simulink model "HW4ThrusterModel"  (R2022b)
settings: Solver=VariableStepAuto  StartTime=0.0  StopTime=20.0  RelTol=1e-3
undefined symbols (not defined in the file or in its folder): sat, trigger, trigger2
settings Model: Creator=gagandeepthapar  LastModifiedBy=gagandeepthapar

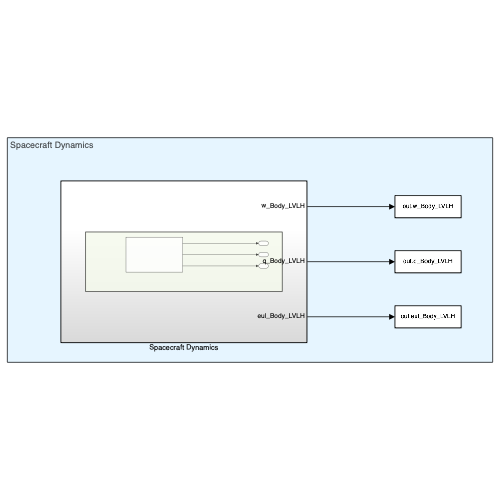
[thumbnail: Simulink's stored preview of the top-level diagram]
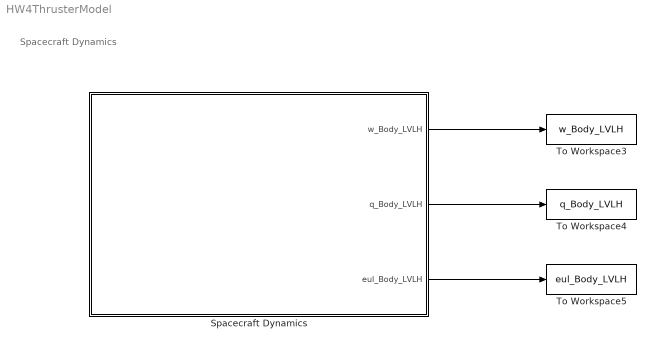
== system HW4ThrusterModel ==
  note: Spacecraft Dynamics
  Spacecraft Dynamics : Subsystem
  To Workspace3 : ToWorkspace  VariableName=w_Body_LVLH  SampleTime=-1
      settings: Save2DSignal=2-D array (concatenate along first dimension)
  To Workspace4 : ToWorkspace  VariableName=q_Body_LVLH  SampleTime=-1
      settings: Save2DSignal=2-D array (concatenate along first dimension)
  To Workspace5 : ToWorkspace  VariableName=eul_Body_LVLH  SampleTime=-1
      settings: Save2DSignal=2-D array (concatenate along first dimension)
  wires:
  Spacecraft Dynamics/1(w_Body_LVLH) -> To Workspace3/1
  Spacecraft Dynamics/2(q_Body_LVLH) -> To Workspace4/1
  Spacecraft Dynamics/3(eul_Body_LVLH) -> To Workspace5/1

== system HW4ThrusterModel/Spacecraft Dynamics ==
  note: Body_LVLH
  Body_LVLH : Subsystem
  w_Body_LVLH : Outport
  q_Body_LVLH : Outport  Port=2
  eul_Body_LVLH : Outport  Port=3
  wires:
  Body_LVLH/1(w_Body_LVLH) -> w_Body_LVLH/1
  Body_LVLH/2(q_Body_LVLH) -> q_Body_LVLH/1
  Body_LVLH/3(eul_Body_LVLH) -> eul_Body_LVLH/1

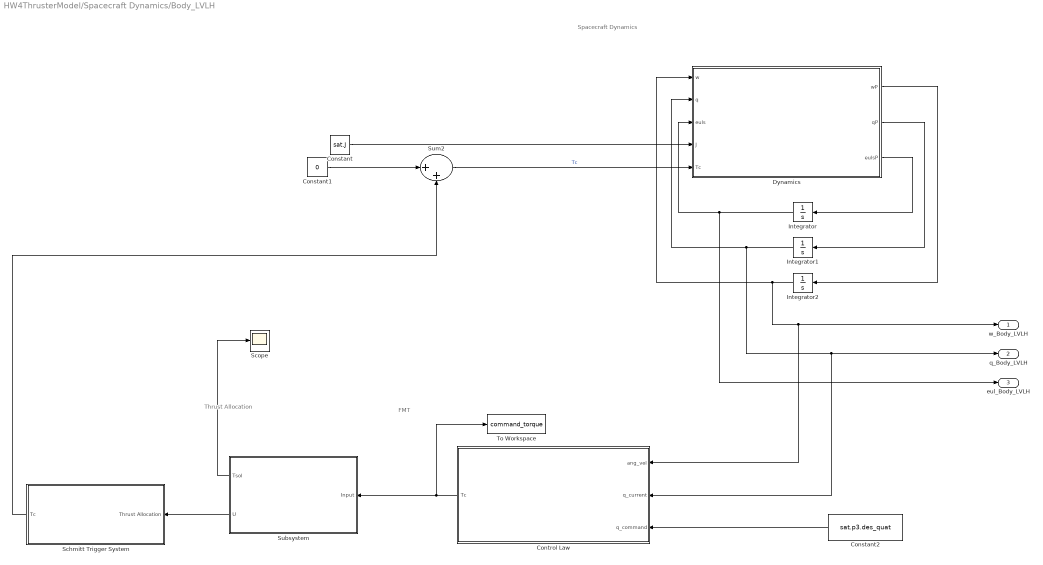
== system HW4ThrusterModel/Spacecraft Dynamics/Body_LVLH ==
  note: Thrust Allocation
  note: Spacecraft Dynamics
  note: FMT
  Constant : Constant  Value=sat.J
  Constant1 : Constant  Value=0
  Constant2 : Constant  Value=sat.p3.des_quat
  Control Law : Subsystem
  Dynamics : MATLAB Function  TreatAsAtomicUnit=on
  Integrator : Integrator  InitialCondition=sat.p3.euls0_lvlh
  Integrator1 : Integrator  InitialCondition=sat.p3.quat0
  Integrator2 : Integrator  InitialCondition=sat.p3.w0_lvlh
  Schmitt Trigger System : Subsystem
  Scope : Scope
  Subsystem : Subsystem
  Sum2 : Sum  Inputs=|++
  To Workspace : ToWorkspace  VariableName=command_torque  SampleTime=-1
      settings: Save2DSignal=2-D array (concatenate along first dimension)
  w_Body_LVLH : Outport
  q_Body_LVLH : Outport  Port=2
  eul_Body_LVLH : Outport  Port=3
  wires:
  Dynamics/3(eulsP) -> Integrator/1
  Dynamics/2(qP) -> Integrator1/1
  Dynamics/1(wP) -> Integrator2/1
  Integrator/1 -> eul_Body_LVLH/1, Dynamics/3(euls)
  Integrator1/1 -> q_Body_LVLH/1, Control Law/2(q_current), Dynamics/2(q)
  Constant/1 -> Dynamics/4(J)
  Constant1/1 -> Sum2/1
  Integrator2/1 -> w_Body_LVLH/1, Control Law/1(ang_vel), Dynamics/1(w)
  Sum2/1 -> Dynamics/5(Tc)  "Tc"
  Control Law/1(Tc) -> To Workspace/1, Subsystem/1(Input)
  Constant2/1 -> Control Law/3(q_command)
  Subsystem/2(U) -> Schmitt Trigger System/1(Thrust Allocation)
  Subsystem/1(Tsol) -> Scope/1
  Schmitt Trigger System/1(Tc) -> Sum2/2

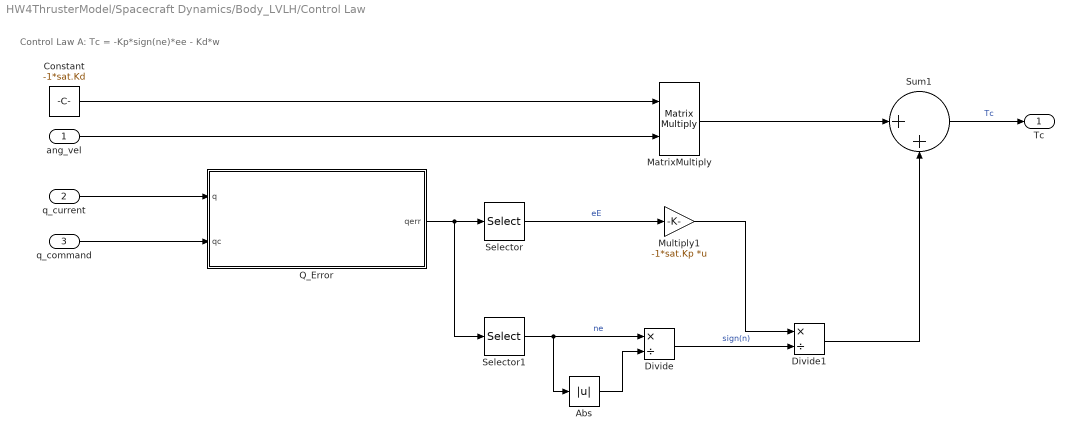
== system HW4ThrusterModel/Spacecraft Dynamics/Body_LVLH/Control Law ==
  note: Control Law A: Tc = -Kp*sign(ne)*ee - Kd*w
  ang_vel : Inport
  q_current : Inport  Port=2
  q_command : Inport  Port=3
  Abs : Abs  SaturateOnIntegerOverflow=off
  Constant : Constant  Value=-1*sat.Kd
  Divide : Product  Inputs=*/
  Divide1 : Product  Inputs=*/
  MatrixMultiply : Product  Multiplication=Matrix(*)
  Multiply1 : Gain  Gain=-1*sat.Kp  Multiplication=Matrix(K*u)
  Q_Error : MATLAB Function  TreatAsAtomicUnit=on
  Selector : Selector  InputPortWidth=4  IndexOptions=Index vector (dialog)  Indices=[1:3]  OutputSizes=1
  Selector1 : Selector  InputPortWidth=4  IndexOptions=Index vector (dialog)  Indices=[4]  OutputSizes=1
  Sum1 : Sum  Inputs=|++
  Tc : Outport
  wires:
  Sum1/1 -> Tc/1  "Tc"
  q_command/1 -> Q_Error/2(qc)
  Abs/1 -> Divide/2
  Selector/1 -> Multiply1/1  "eE"
  Divide/1 -> Divide1/2  "sign(n)"
  Selector1/1 -> Divide/1, Abs/1  "ne"
  q_current/1 -> Q_Error/1(q)
  Multiply1/1 -> Divide1/1
  Q_Error/1(qerr) -> Selector/1, Selector1/1
  Divide1/1 -> Sum1/2
  MatrixMultiply/1 -> Sum1/1
  Constant/1 -> MatrixMultiply/1
  ang_vel/1 -> MatrixMultiply/2

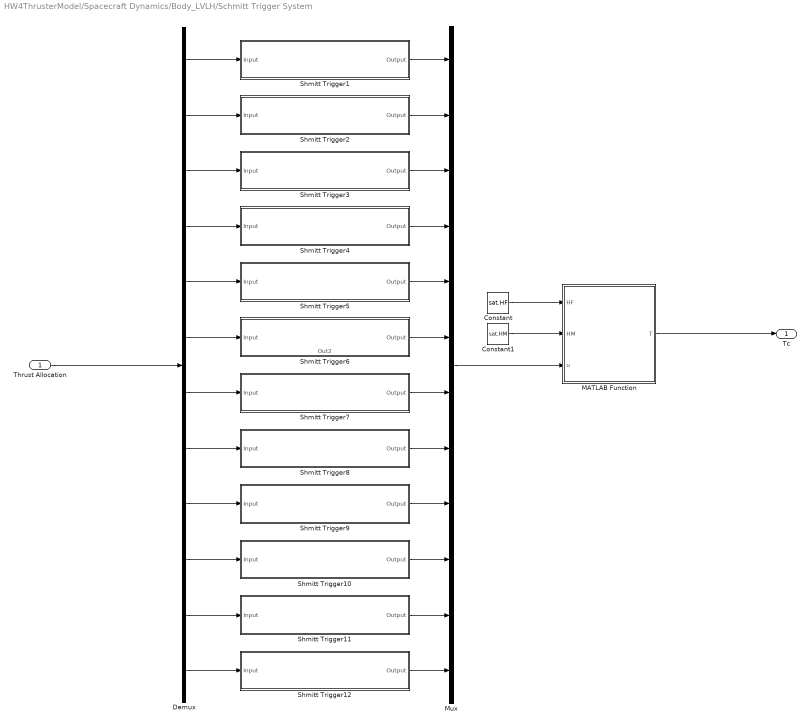
== system HW4ThrusterModel/Spacecraft Dynamics/Body_LVLH/Schmitt Trigger System ==
  Thrust Allocation : Inport
  Constant : Constant  Value=sat.HF
  Constant1 : Constant  Value=sat.HM
  Demux : Demux  Outputs=12
  MATLAB Function : MATLAB Function  TreatAsAtomicUnit=on
  Mux : Mux  Inputs=12
  Shmitt Trigger1 : Subsystem
  Shmitt Trigger10 : Subsystem
  Shmitt Trigger11 : Subsystem
  Shmitt Trigger12 : Subsystem
  Shmitt Trigger2 : Subsystem
  Shmitt Trigger3 : Subsystem
  Shmitt Trigger4 : Subsystem
  Shmitt Trigger5 : Subsystem
  Shmitt Trigger6 : Subsystem
      settings: PortSchema="{\"entries\":[{\"content\":{\"sides\":[{\"content\":{\"connectorIds\":[\"In1\"]},\"type\":\"ConnectorPlacement.EquallySpacedRectSide\",\"uuid\":\"5267026c-02ab-4f60-88ae-288709194649\"},{\"content\":{\"connectorIds\":[\"Out1\"],\"side\":\"RIGHT\"},\"type\":\"ConnectorPlacement.EquallySpacedRectSide\",\"uuid\":\"e9b9484e-3766-44b2-b9f0-a66efab5cfe3\"},{\"content\":{\"connectorIds\":[],\"side\":\"TOP\"},\"type\":\"ConnectorPlacement.EquallySpacedRectSide\",\"uuid\":\"dcb3a7da-9379-4c65-a8d2-aa3203b60853\"},{\"content\":{\"connectorIds\":[\"Out2\"],\"side\":\"BOTTOM\"},\"type\":\"ConnectorPlacement.EquallySpacedRectSide\",\"uuid\":\"f7a7aea4-334d-4b94-b9b6-9901d8a0050a\"}]},\"type\":\"ConnectorPlacement.EquallySpacedConnector\",\"uuid\":\"fe3f15dc-b3d8-4001-8bf5-6903a8817469\"}],\"packageUris\":[\"http://schema.mathworks.com/mf0/Connector/R2020b\"],\"version\":\"1.0\"}"
  Shmitt Trigger7 : Subsystem
  Shmitt Trigger8 : Subsystem
  Shmitt Trigger9 : Subsystem
  Tc : Outport
  wires:
  Thrust Allocation/1 -> Demux/1
  Demux/1 -> Shmitt Trigger1/1(Input)
  Shmitt Trigger1/1(Output) -> Mux/1
  Shmitt Trigger2/1(Output) -> Mux/2
  Demux/2 -> Shmitt Trigger2/1(Input)
  Demux/3 -> Shmitt Trigger3/1(Input)
  Shmitt Trigger3/1(Output) -> Mux/3
  Demux/4 -> Shmitt Trigger4/1(Input)
  Shmitt Trigger4/1(Output) -> Mux/4
  Demux/5 -> Shmitt Trigger5/1(Input)
  Demux/6 -> Shmitt Trigger6/1(Input)
  Demux/7 -> Shmitt Trigger7/1(Input)
  Demux/8 -> Shmitt Trigger8/1(Input)
  Demux/9 -> Shmitt Trigger9/1(Input)
  Demux/10 -> Shmitt Trigger10/1(Input)
  Demux/11 -> Shmitt Trigger11/1(Input)
  Demux/12 -> Shmitt Trigger12/1(Input)
  Shmitt Trigger12/1(Output) -> Mux/12
  Shmitt Trigger11/1(Output) -> Mux/11
  Shmitt Trigger10/1(Output) -> Mux/10
  Shmitt Trigger9/1(Output) -> Mux/9
  Shmitt Trigger8/1(Output) -> Mux/8
  Shmitt Trigger7/1(Output) -> Mux/7
  Shmitt Trigger6/1(Output) -> Mux/6
  Shmitt Trigger5/1(Output) -> Mux/5
  Mux/1 -> MATLAB Function/3(u)
  Constant/1 -> MATLAB Function/1(HF)
  Constant1/1 -> MATLAB Function/2(HM)
  MATLAB Function/1(T) -> Tc/1

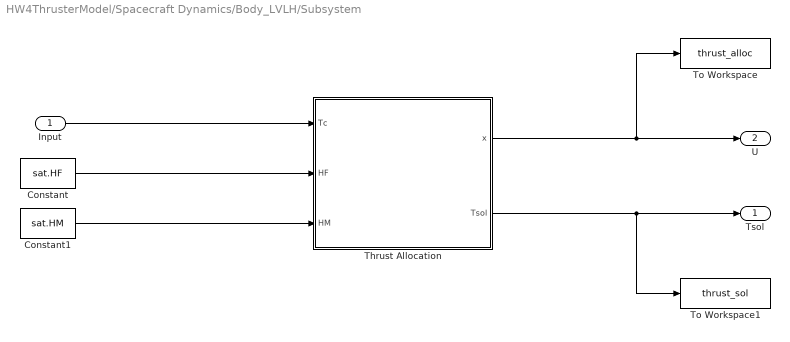
== system HW4ThrusterModel/Spacecraft Dynamics/Body_LVLH/Subsystem ==
  Input : Inport
  Constant : Constant  Value=sat.HF
  Constant1 : Constant  Value=sat.HM
  Thrust Allocation : MATLAB Function  TreatAsAtomicUnit=on
  To Workspace : ToWorkspace  VariableName=thrust_alloc  SampleTime=-1
      settings: Save2DSignal=2-D array (concatenate along first dimension)
  To Workspace1 : ToWorkspace  VariableName=thrust_sol  SampleTime=-1
      settings: Save2DSignal=2-D array (concatenate along first dimension)
  Tsol : Outport  PortDimensions=[3 1]
  U : Outport  Port=2  PortDimensions=[12 1]
  wires:
  Constant/1 -> Thrust Allocation/2(HF)
  Constant1/1 -> Thrust Allocation/3(HM)
  Thrust Allocation/2(Tsol) -> To Workspace1/1, Tsol/1
  Thrust Allocation/1(x) -> U/1, To Workspace/1
  Input/1 -> Thrust Allocation/1(Tc)

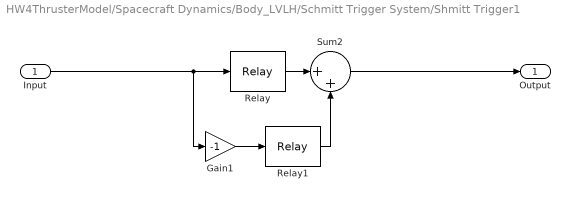
== system HW4ThrusterModel/Spacecraft Dynamics/Body_LVLH/Schmitt Trigger System/Shmitt Trigger1 ==
  Input : Inport
  Gain1 : Gain  Gain=-1
  Relay : Relay  OnSwitchValue=trigger2.delOn  OffSwitchValue=trigger2.delOff  OnOutputValue=trigger.mag  ZeroCross=off
  Relay1 : Relay  OnSwitchValue=trigger2.delOn  OffSwitchValue=trigger2.delOff  OnOutputValue=-1*trigger.mag  ZeroCross=off
  Sum2 : Sum  Inputs=|++
  Output : Outport
  wires:
  Gain1/1 -> Relay1/1
  Input/1 -> Gain1/1, Relay/1
  Relay/1 -> Sum2/1
  Relay1/1 -> Sum2/2
  Sum2/1 -> Output/1

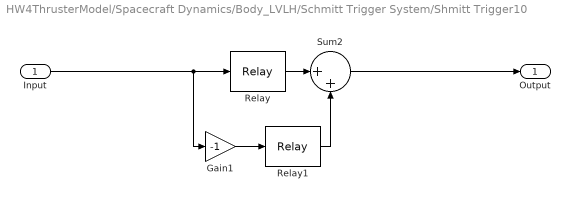
== system HW4ThrusterModel/Spacecraft Dynamics/Body_LVLH/Schmitt Trigger System/Shmitt Trigger10 ==
  Input : Inport
  Gain1 : Gain  Gain=-1
  Relay : Relay  OnSwitchValue=trigger2.delOn  OffSwitchValue=trigger2.delOff  OnOutputValue=trigger.mag  ZeroCross=off
  Relay1 : Relay  OnSwitchValue=trigger2.delOn  OffSwitchValue=trigger2.delOff  OnOutputValue=-1*trigger.mag  ZeroCross=off
  Sum2 : Sum  Inputs=|++
  Output : Outport
  wires:
  Gain1/1 -> Relay1/1
  Input/1 -> Gain1/1, Relay/1
  Relay/1 -> Sum2/1
  Relay1/1 -> Sum2/2
  Sum2/1 -> Output/1

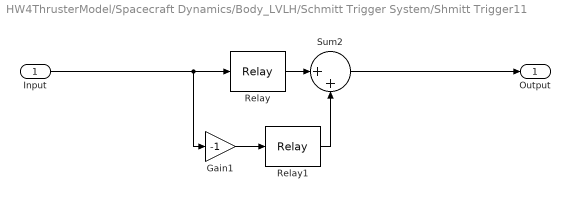
== system HW4ThrusterModel/Spacecraft Dynamics/Body_LVLH/Schmitt Trigger System/Shmitt Trigger11 ==
  Input : Inport
  Gain1 : Gain  Gain=-1
  Relay : Relay  OnSwitchValue=trigger2.delOn  OffSwitchValue=trigger2.delOff  OnOutputValue=trigger.mag  ZeroCross=off
  Relay1 : Relay  OnSwitchValue=trigger2.delOn  OffSwitchValue=trigger2.delOff  OnOutputValue=-1*trigger.mag  ZeroCross=off
  Sum2 : Sum  Inputs=|++
  Output : Outport
  wires:
  Gain1/1 -> Relay1/1
  Input/1 -> Gain1/1, Relay/1
  Relay/1 -> Sum2/1
  Relay1/1 -> Sum2/2
  Sum2/1 -> Output/1

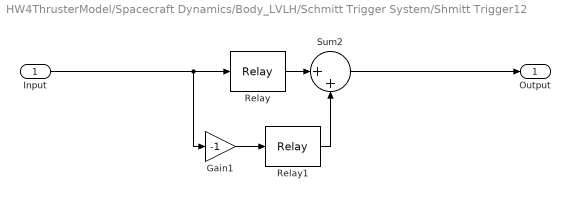
== system HW4ThrusterModel/Spacecraft Dynamics/Body_LVLH/Schmitt Trigger System/Shmitt Trigger12 ==
  Input : Inport
  Gain1 : Gain  Gain=-1
  Relay : Relay  OnSwitchValue=trigger2.delOn  OffSwitchValue=trigger2.delOff  OnOutputValue=trigger.mag  ZeroCross=off
  Relay1 : Relay  OnSwitchValue=trigger2.delOn  OffSwitchValue=trigger2.delOff  OnOutputValue=-1*trigger.mag  ZeroCross=off
  Sum2 : Sum  Inputs=|++
  Output : Outport
  wires:
  Gain1/1 -> Relay1/1
  Input/1 -> Gain1/1, Relay/1
  Relay/1 -> Sum2/1
  Relay1/1 -> Sum2/2
  Sum2/1 -> Output/1

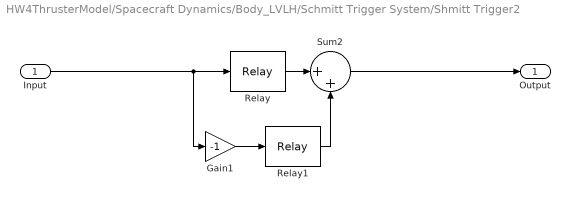
== system HW4ThrusterModel/Spacecraft Dynamics/Body_LVLH/Schmitt Trigger System/Shmitt Trigger2 ==
  Input : Inport
  Gain1 : Gain  Gain=-1
  Relay : Relay  OnSwitchValue=trigger2.delOn  OffSwitchValue=trigger2.delOff  OnOutputValue=trigger.mag  ZeroCross=off
  Relay1 : Relay  OnSwitchValue=trigger2.delOn  OffSwitchValue=trigger2.delOff  OnOutputValue=-1*trigger.mag  ZeroCross=off
  Sum2 : Sum  Inputs=|++
  Output : Outport
  wires:
  Gain1/1 -> Relay1/1
  Input/1 -> Gain1/1, Relay/1
  Relay/1 -> Sum2/1
  Relay1/1 -> Sum2/2
  Sum2/1 -> Output/1

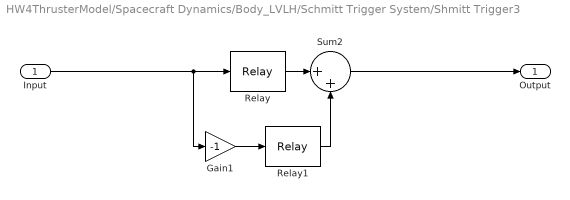
== system HW4ThrusterModel/Spacecraft Dynamics/Body_LVLH/Schmitt Trigger System/Shmitt Trigger3 ==
  Input : Inport
  Gain1 : Gain  Gain=-1
  Relay : Relay  OnSwitchValue=trigger2.delOn  OffSwitchValue=trigger2.delOff  OnOutputValue=trigger.mag  ZeroCross=off
  Relay1 : Relay  OnSwitchValue=trigger2.delOn  OffSwitchValue=trigger2.delOff  OnOutputValue=-1*trigger.mag  ZeroCross=off
  Sum2 : Sum  Inputs=|++
  Output : Outport
  wires:
  Gain1/1 -> Relay1/1
  Input/1 -> Gain1/1, Relay/1
  Relay/1 -> Sum2/1
  Relay1/1 -> Sum2/2
  Sum2/1 -> Output/1

== system HW4ThrusterModel/Spacecraft Dynamics/Body_LVLH/Schmitt Trigger System/Shmitt Trigger4 ==
  Input : Inport
  Gain1 : Gain  Gain=-1
  Relay : Relay  OnSwitchValue=trigger2.delOn  OffSwitchValue=trigger2.delOff  OnOutputValue=trigger.mag  ZeroCross=off
  Relay1 : Relay  OnSwitchValue=trigger2.delOn  OffSwitchValue=trigger2.delOff  OnOutputValue=-1*trigger.mag  ZeroCross=off
  Sum2 : Sum  Inputs=|++
  Output : Outport
  wires:
  Gain1/1 -> Relay1/1
  Input/1 -> Gain1/1, Relay/1
  Relay/1 -> Sum2/1
  Relay1/1 -> Sum2/2
  Sum2/1 -> Output/1

== system HW4ThrusterModel/Spacecraft Dynamics/Body_LVLH/Schmitt Trigger System/Shmitt Trigger5 ==
  Input : Inport
  Gain1 : Gain  Gain=-1
  Relay : Relay  OnSwitchValue=trigger2.delOn  OffSwitchValue=trigger2.delOff  OnOutputValue=trigger.mag  ZeroCross=off
  Relay1 : Relay  OnSwitchValue=trigger2.delOn  OffSwitchValue=trigger2.delOff  OnOutputValue=-1*trigger.mag  ZeroCross=off
  Sum2 : Sum  Inputs=|++
  Output : Outport
  wires:
  Gain1/1 -> Relay1/1
  Input/1 -> Gain1/1, Relay/1
  Relay/1 -> Sum2/1
  Relay1/1 -> Sum2/2
  Sum2/1 -> Output/1

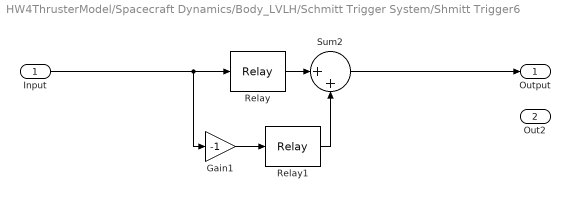
== system HW4ThrusterModel/Spacecraft Dynamics/Body_LVLH/Schmitt Trigger System/Shmitt Trigger6 ==
  Input : Inport
  Gain1 : Gain  Gain=-1
  Relay : Relay  OnSwitchValue=trigger2.delOn  OffSwitchValue=trigger2.delOff  OnOutputValue=trigger.mag  ZeroCross=off
  Relay1 : Relay  OnSwitchValue=trigger2.delOn  OffSwitchValue=trigger2.delOff  OnOutputValue=-1*trigger.mag  ZeroCross=off
  Sum2 : Sum  Inputs=|++
  Output : Outport
  Out2 : Outport  Port=2
  wires:
  Gain1/1 -> Relay1/1
  Input/1 -> Gain1/1, Relay/1
  Relay/1 -> Sum2/1
  Relay1/1 -> Sum2/2
  Sum2/1 -> Output/1

== system HW4ThrusterModel/Spacecraft Dynamics/Body_LVLH/Schmitt Trigger System/Shmitt Trigger7 ==
  Input : Inport
  Gain1 : Gain  Gain=-1
  Relay : Relay  OnSwitchValue=trigger2.delOn  OffSwitchValue=trigger2.delOff  OnOutputValue=trigger.mag  ZeroCross=off
  Relay1 : Relay  OnSwitchValue=trigger2.delOn  OffSwitchValue=trigger2.delOff  OnOutputValue=-1*trigger.mag  ZeroCross=off
  Sum2 : Sum  Inputs=|++
  Output : Outport
  wires:
  Gain1/1 -> Relay1/1
  Input/1 -> Gain1/1, Relay/1
  Relay/1 -> Sum2/1
  Relay1/1 -> Sum2/2
  Sum2/1 -> Output/1

== system HW4ThrusterModel/Spacecraft Dynamics/Body_LVLH/Schmitt Trigger System/Shmitt Trigger8 ==
  Input : Inport
  Gain1 : Gain  Gain=-1
  Relay : Relay  OnSwitchValue=trigger2.delOn  OffSwitchValue=trigger2.delOff  OnOutputValue=trigger.mag  ZeroCross=off
  Relay1 : Relay  OnSwitchValue=trigger2.delOn  OffSwitchValue=trigger2.delOff  OnOutputValue=-1*trigger.mag  ZeroCross=off
  Sum2 : Sum  Inputs=|++
  Output : Outport
  wires:
  Gain1/1 -> Relay1/1
  Input/1 -> Gain1/1, Relay/1
  Relay/1 -> Sum2/1
  Relay1/1 -> Sum2/2
  Sum2/1 -> Output/1

== system HW4ThrusterModel/Spacecraft Dynamics/Body_LVLH/Schmitt Trigger System/Shmitt Trigger9 ==
  Input : Inport
  Gain1 : Gain  Gain=-1
  Relay : Relay  OnSwitchValue=trigger2.delOn  OffSwitchValue=trigger2.delOff  OnOutputValue=trigger.mag  ZeroCross=off
  Relay1 : Relay  OnSwitchValue=trigger2.delOn  OffSwitchValue=trigger2.delOff  OnOutputValue=-1*trigger.mag  ZeroCross=off
  Sum2 : Sum  Inputs=|++
  Output : Outport
  wires:
  Gain1/1 -> Relay1/1
  Input/1 -> Gain1/1, Relay/1
  Relay/1 -> Sum2/1
  Relay1/1 -> Sum2/2
  Sum2/1 -> Output/1

== matlab function HW4ThrusterModel/Spacecraft Dynamics/Body_LVLH/Schmitt Trigger System/MATLAB Function ==
  data: HF input; HM input; u input; T output
function T = fcn(HF, HM, u)

H = [HF;HM];
T = HM*u;

== matlab function HW4ThrusterModel/Spacecraft Dynamics/Body_LVLH/Subsystem/Thrust Allocation ==
  data: Tc input size=[3 1]; x output size=[12 1]; HF input size=[3 12]; Tsol output size=[3 1]; HM input size=[3 12]
function [x, Tsol] = fcn(Tc, HF, HM)

coder.extrinsic('linprog');
coder.extrinsic('intlinprog');
coder.extrinsic('optimoptions')

intlinprogflag = 0;

x = zeros(12,1);
lb = zeros(12,1);   % lower bound
ub = 50 * ones(12,1);   % upper bound
f = ones(1,12); % cost function to minimize is the sum of all thrusters

translate_sol = zeros(3,1); % want 0 translation
moment_sol = Tc;    % need to reach ideal Tc using thruster alloc

H = [HF;HM];    % combine translate/moment matrices

%Aeq = H;    % allocation matrix
Aeq = HM;

%Beq = [translate_sol;moment_sol]; % solution matrix
Beq = moment_sol;



if intlinprogflag == 1
    intcon = 1:12;
    options = optimoptions('intlinprog', 'Display', 'off');
    x = intlinprog(f, intcon, [], [], Aeq, Beq,  lb, ub, [], options);   % solves linprog problem

else
    options = optimoptions('linprog', 'Display', 'off');
    x = linprog(f, [], [], Aeq, Beq, lb, ub, options);

    % using least squares method
    %x = inv(Aeq'*Aeq)*(Aeq'*Beq);

end

Tsol = Aeq * x;












Tsol = HM*x;    % gets torque from thruster allocation

== matlab function HW4ThrusterModel/Spacecraft Dynamics/Body_LVLH/Dynamics ==
  data: w input; q input; euls input; wP output; J input; Tc input; qP output; eulsP output
function [wP, qP, eulsP] = fcn(w, q, euls, J, Tc)
    
    function wx = skewSymmetric(w)
        wx = [0, -1*w(3), w(2);
             w(3), 0, -1*w(1);
             -1*w(2), w(1), 0];
    end

    T = [Tc(1);Tc(2);Tc(3)];

    wP = J\(T - skewSymmetric(w)*J*w);

    e = q(1:3);
    n = q(4);
    eP = 0.5*(n*eye(3) + skewSymmetric(e))*w;
    nP = -0.5*e'*w;
    qP = [eP;nP];

    phi = euls(1);
    theta = euls(2);
    psi = euls(3);
    eulsP = 1/(cos(theta)) * [cos(theta), sin(phi)*sin(theta), cos(phi)*sin(theta);
                                0, cos(phi)*cos(theta), -1*sin(phi)*cos(theta);
                                0, sin(phi), cos(phi)] * w;


end

== matlab function HW4ThrusterModel/Spacecraft Dynamics/Body_LVLH/Control Law/Q_Error ==
  data: q input; qerr output; qc input
function qerr = fcn(q, qc)

%     function wx = skewSymmetric(w)
%         wx = [0, -1*w(3), w(2);
%              w(3), 0, -1*w(1);
%              -1*w(2), w(1), 0];
%     end

    function qp = quatmult(q, p)
    
        function wx = skewSymmetric(w)
            wx = [0, -1*w(3), w(2);
                 w(3), 0, -1*w(1);
                 -1*w(2), w(1), 0];
        end
    
        qn = q(4);
        qe = q(1:3);
    
        pn = p(4);
        pe = p(1:3);
    
        n = pn * qn - pe'*qe;
        e = pn * qe + qn*pe + skewSymmetric(pe)*qe;
    
        qp = [e(1);e(2);e(3);n];
    
    end

qc(1:3) = -1*qc(1:3);
qerr = quatmult(qc, q);

end
